simulink model "FSK1"  (R2015a)
settings: Solver=ode45  StartTime=0.0  StopTime=10.0  RelTol=1e-3
libraries: commdigbbndfm2 x2, commchan3 x1, commsink2 x1, commrandsrc2 x1
settings Model: Creator=Lenovo  LastModifiedBy=Lenovo

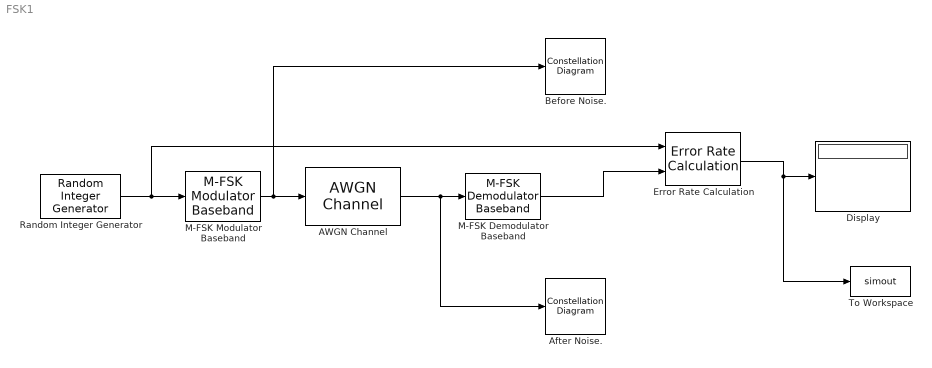
== system FSK1 ==
  AWGN Channel : commchan3/AWGN Channel  InputProcessing=Columns as channels (frame based)  seed=67  noiseMode="Signal to noise ratio  (Eb/No)"  EbNodB=EbNo  EsNodB=10  SNRdB=10  bitsPerSym=3  Ps=1  Tsym=1  variance=1
  "After Noise. " : ConstellationDiagram
  Before Noise. : ConstellationDiagram
  Display : Display
  Error Rate Calculation : commsink2/Error Rate Calculation  N=0  st_delay=0  cp_mode=Entire frame  subframe=[]  PMode=Port  WsName=ErrorVec  RsMode2=off  stop=off  numErr=100  maxBits=1e6
  M-FSK Demodulator Baseband : commdigbbndfm2/M-FSK Demodulator Baseband  M=8  OutType=Integer  Dec=Binary  freqSep=6  numSamp=17  RateOptions=Enforce single-rate processing  outDataType=double
  M-FSK Modulator Baseband : commdigbbndfm2/M-FSK Modulator Baseband  M=8  InType=Integer  Enc=Binary  freqSep=6  phaseType=Continuous  numSamp=17  RateOptions=Enforce single-rate processing  outDataType=double
  Random Integer Generator : commrandsrc2/Random Integer Generator  mul=8  seed=37  Ts=1  frameBased=on  sampPerFrame=100  orient=off  outDataType=double
  To Workspace : ToWorkspace  VariableName=simout  SampleTime=-1
      settings: Save2DSignal=2-D array (concatenate along first dimension)
  wires:
  Error Rate Calculation/1 -> Display/1, To Workspace/1
  Random Integer Generator/1 -> M-FSK Modulator Baseband/1, Error Rate Calculation/1
  AWGN Channel/1 -> M-FSK Demodulator Baseband/1, "After Noise. "/1
  M-FSK Modulator Baseband/1 -> AWGN Channel/1, Before Noise./1
  M-FSK Demodulator Baseband/1 -> Error Rate Calculation/2
